simulink model "lab21__1"  (R2018b)
settings: Solver=VariableStepAuto  StartTime=0.0  StopTime=10.0  RelTol=1e-3
undefined symbols (not defined in the file): b, f, k, m
settings Model: Creator=student  LastModifiedBy=student

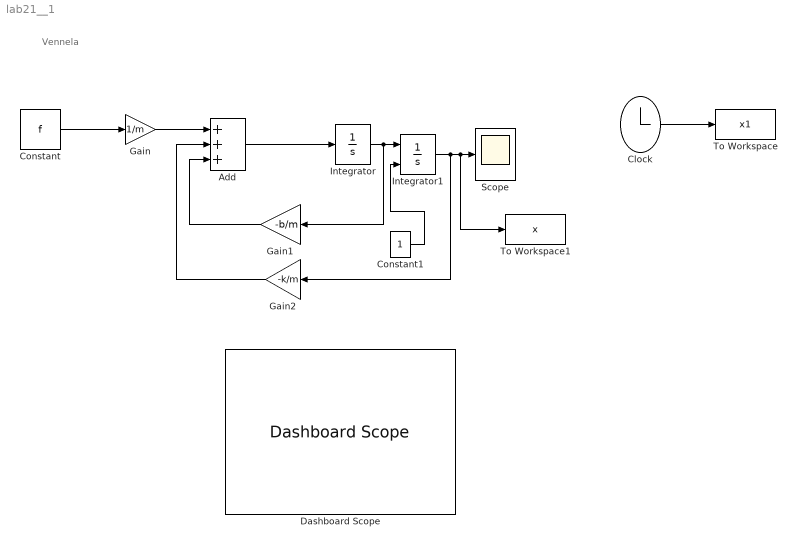
== system lab21__1 ==
  note: Vennela
  Add : Sum  Inputs=+++
  Clock : Clock
  Constant : Constant  Value=f  VectorParams1D=off  SampleTime=-1
  Constant1 : Constant
  Dashboard Scope : DashboardScope  WebBlockId=15
  Gain : Gain  Gain=1/m
  Gain1 : Gain  Gain=-b/m
  Gain2 : Gain  Gain=-k/m
  Integrator : Integrator
  Integrator1 : Integrator  InitialConditionSource=external
  Scope : Scope
  To Workspace : ToWorkspace  VariableName=x1  SampleTime=-1
  To Workspace1 : ToWorkspace  VariableName=x  SampleTime=-1
  wires:
  Constant/1 -> Gain/1
  Gain/1 -> Add/1
  Gain1/1 -> Add/3
  Gain2/1 -> Add/2
  Integrator/1 -> Gain1/1, Integrator1/1
  Integrator1/1 -> To Workspace1/1, Scope/1, Gain2/1
  Add/1 -> Integrator/1
  Clock/1 -> To Workspace/1
  Constant1/1 -> Integrator1/2
